simulink model "Feedback_Configuration_1"  (R2022a)
settings: Solver=VariableStepAuto  StartTime=0.0  StopTime=300  RelTol=1e-3
libraries: cstblocks x3
settings Model: Creator=User  LastModifiedBy=User

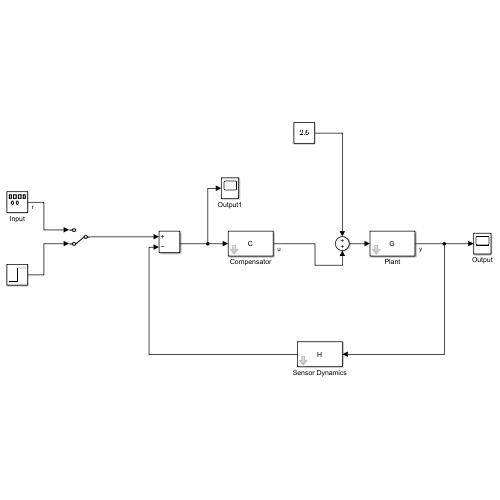
[thumbnail: Simulink's stored preview of the top-level diagram]
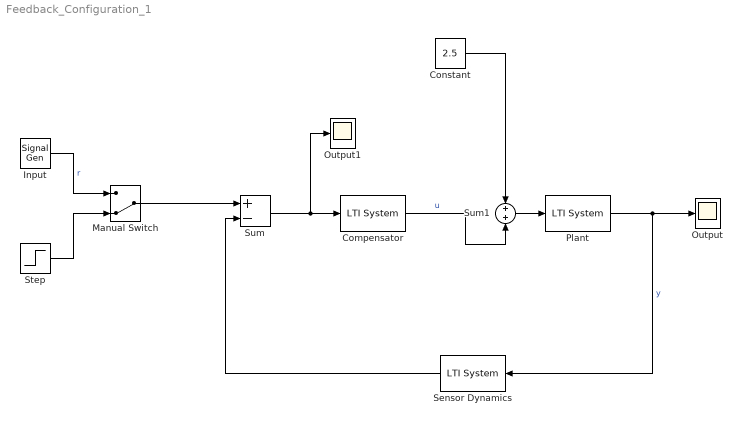
== system Feedback_Configuration_1 ==
  Compensator : cstblocks/LTI System  sys=C  IC=[]
  Constant : Constant  Value=2.5  SampleTime=-1
  Input : SignalGenerator
  Manual Switch : ManualSwitch  CurrentSetting=0
  Output : Scope
  Output1 : Scope
  Plant : cstblocks/LTI System  sys=G  IC=[]
  Sensor Dynamics : cstblocks/LTI System  sys=H  IC=[]
  Step : Step  Before=2.5  After=5  SampleTime=0
  Sum : Sum  Inputs=+-
  Sum1 : Sum  Inputs=+|+
  wires:
  Manual Switch/1 -> Sum/1
  Sensor Dynamics/1 -> Sum/2
  Sum/1 -> Output1/1, Compensator/1
  Plant/1 -> Output/1, Sensor Dynamics/1  "y"
  Input/1 -> Manual Switch/1  "r"
  Step/1 -> Manual Switch/2
  Constant/1 -> Sum1/1
  Sum1/1 -> Plant/1
  Compensator/1 -> Sum1/2  "u"
